simulink library "libMdl_transpQuat"  (R2018a)
settings: Solver=VariableStepAuto  StartTime=0.0  StopTime=10.0  RelTol=1e-3
settings Model: Creator=hwinter  LastModifiedBy=Hanno

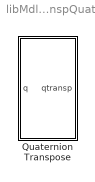
== system libMdl_transpQuat ==
  Quaternion Transpose : Subsystem
      mask Display:
      | color('black')
      | port_label('input', 1, 'q', 'texmode','on')
      | port_label('output', 1, 'q''', 'texmode','on')

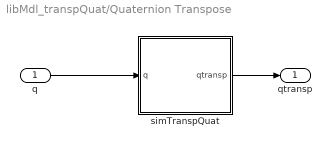
== system libMdl_transpQuat/Quaternion Transpose ==
  q : Inport
  simTranspQuat : MATLAB Function  TreatAsAtomicUnit=on
  qtransp : Outport
  wires:
  q/1 -> simTranspQuat/1(q)
  simTranspQuat/1(qtransp) -> qtransp/1

== matlab function libMdl_transpQuat/Quaternion Transpose/simTranspQuat ==
  data: q input; qtransp output
function qtransp = simTranspQuat(q)

qtransp = transpQuat(q);

end % function
